simulink model "SeptimoBSimulink"  (R2017b)
settings: Solver=VariableStepAuto  StartTime=0.0  StopTime=20  RelTol=1e-3
values from neighbouring files (symbols this model uses):
  kd = eval(S.kd)    [Cuarto_P_I_D.m]    (also in Quinto_P_I_D.m; Segundoo.m; SeptimoBPIDD2.m; SeptimoPIDD2.m)
  kd2 = eval(S.kd2)    [Quinto_P_I_D.m]    (also in SeptimoBPIDD2.m; SeptimoPIDD2.m)
  ki = eval(S.ki)    [Cuarto_P_I_D.m]    (also in Quinto_P_I_D.m; Segundoo.m; SeptimoBPIDD2.m; SeptimoPIDD2.m)
  kp = eval(S.kp)    [Cuarto_P_I_D.m]    (also in Quinto_P_I_D.m; Segundoo.m; SeptimoBPIDD2.m; SeptimoPIDD2.m)
settings Model: Creator=Cx001la  LastModifiedBy=Cx001la

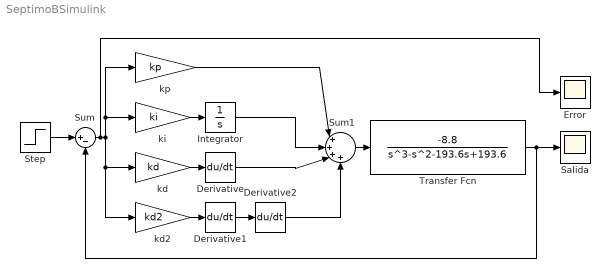
== system SeptimoBSimulink ==
  Derivative : Derivative
  Derivative1 : Derivative
  Derivative2 : Derivative
  Error : Scope
  Integrator : Integrator
  Salida : Scope
  Step : Step  Time=0  SampleTime=0
  Sum : Sum  Inputs=|+-
  Sum1 : Sum  Inputs=|++++
  Transfer Fcn : TransferFcn  Numerator=[-8.8]  Denominator=[1 -1 -193.6 193.6]
  kd : Gain  Gain=kd
  kd2 : Gain  Gain=kd2
  ki : Gain  Gain=ki
  kp : Gain  Gain=kp
  wires:
  ki/1 -> Integrator/1
  Derivative1/1 -> Derivative2/1
  Derivative2/1 -> Sum1/4
  Sum1/1 -> Transfer Fcn/1
  kd2/1 -> Derivative1/1
  Integrator/1 -> Sum1/2
  Transfer Fcn/1 -> Salida/1, Sum/2
  kp/1 -> Sum1/1
  Sum/1 -> Error/1, kp/1, ki/1, kd2/1, kd/1
  Derivative/1 -> Sum1/3
  Step/1 -> Sum/1
  kd/1 -> Derivative/1
